simulink model "lab2q4blockdiagram"  (Simulink 8.7)
settings: Solver=ode45  StartTime=0.0  StopTime=60  RelTol=1e-3
settings Model: Creator=gmcma  LastModifiedBy=gmcma
settings DataIOCC: LimitDataPoints=off  SaveFormat=Dataset
settings DebuggingCC: UnderspecifiedInitializationDetection=Simplified  MergeDetectMultiDrivingBlocksExec=error
settings HardwareCC: ProdBitPerPointer=64  ProdLargestAtomicFloat=Float  ProdIntDivRoundTo=Zero  ProdEndianess=LittleEndian  ProdWordSize=64  ProdHWDeviceType=Intel->x86-64 (Windows64)
settings ModelReferenceCC: PropagateSignalLabelsOutOfModel=on
settings ConfigComp: CovModelRefEnable=off

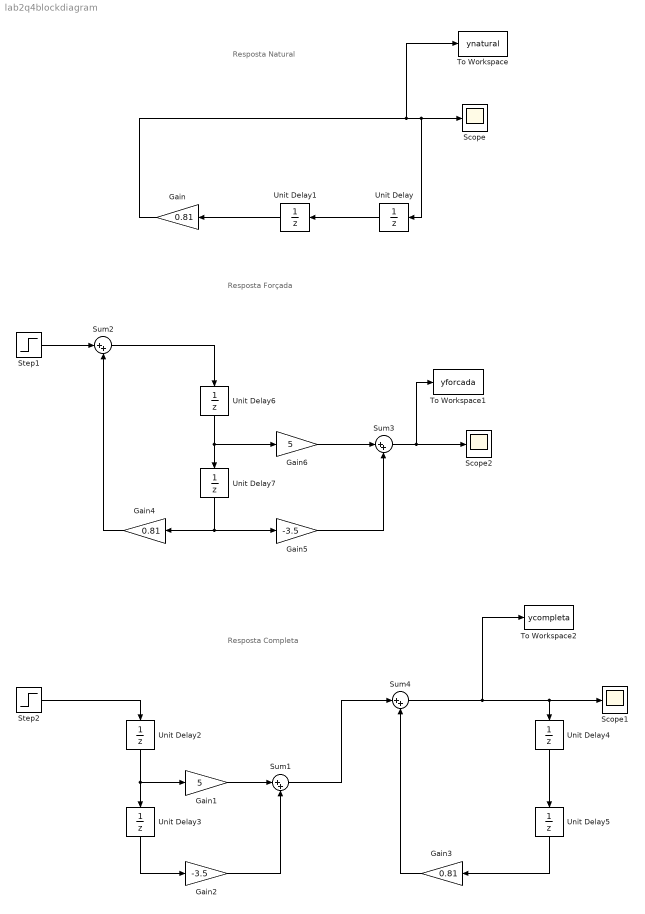
== system lab2q4blockdiagram ==
  note: Resposta Natural
  note: Resposta Forçada
  note: Resposta Completa
  Gain : Gain  Gain=0.81
  Gain1 : Gain  Gain=5
  Gain2 : Gain  Gain=-3.5
  Gain3 : Gain  Gain=0.81
  Gain4 : Gain  Gain=0.81
  Gain5 : Gain  Gain=-3.5
  Gain6 : Gain  Gain=5
  Scope : Scope
  Scope1 : Scope
  Scope2 : Scope
  Step1 : Step  SampleTime=1  ZeroCross=off
  Step2 : Step  SampleTime=1  ZeroCross=off
  Sum{1..4} (4 alike) : Sum  Inputs=|++
  To Workspace : ToWorkspace  VariableName=ynatural  SaveFormat=Structure With Time  SampleTime=-1
  To Workspace1 : ToWorkspace  VariableName=yforcada  SaveFormat=Structure  SampleTime=-1
  To Workspace2 : ToWorkspace  VariableName=ycompleta  SaveFormat=Structure  SampleTime=-1
  Unit Delay : UnitDelay  InitialCondition=-8
  Unit Delay1 : UnitDelay  InitialCondition=-2
  Unit Delay{2..3,6..7} (4 alike) : UnitDelay
  Unit Delay4 : UnitDelay  InitialCondition=-1.6200
  Unit Delay5 : UnitDelay  InitialCondition=-1.4800
  wires:
  Unit Delay/1 -> Unit Delay1/1
  Unit Delay1/1 -> Gain/1
  Step1/1 -> Sum2/1
  Unit Delay7/1 -> Gain4/1, Gain5/1
  Gain4/1 -> Sum2/2
  Unit Delay6/1 -> Gain6/1, Unit Delay7/1
  Sum2/1 -> Unit Delay6/1
  Gain5/1 -> Sum3/2
  Gain6/1 -> Sum3/1
  Sum3/1 -> To Workspace1/1, Scope2/1
  Gain/1 -> To Workspace/1, Scope/1, Unit Delay/1
  Unit Delay2/1 -> Gain1/1, Unit Delay3/1
  Step2/1 -> Unit Delay2/1
  Unit Delay3/1 -> Gain2/1
  Gain2/1 -> Sum1/2
  Gain1/1 -> Sum1/1
  Unit Delay4/1 -> Unit Delay5/1
  Unit Delay5/1 -> Gain3/1
  Gain3/1 -> Sum4/2
  Sum1/1 -> Sum4/1
  Sum4/1 -> To Workspace2/1, Scope1/1, Unit Delay4/1
